simulink model "control_velocidades"  (Simulink 7.5)
settings: Solver=ode45  StartTime=0.0  StopTime=10.0  RelTol=1e-3
libraries: simulink x1
settings Model: Creator=ARTURO  LastModifiedBy=ARTURO

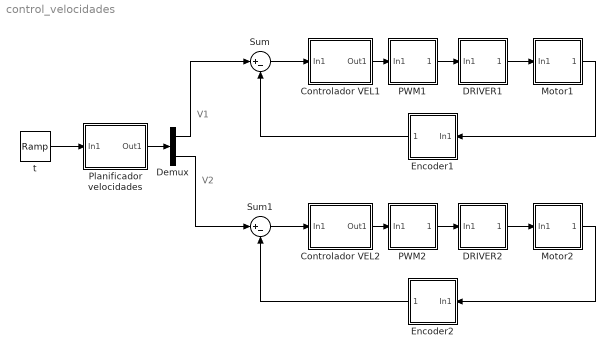
== system control_velocidades ==
  note: V1
  note: V2
  Controlador VEL1 : Subsystem
  Controlador VEL2 : Subsystem
  DRIVER1 : Subsystem
  DRIVER2 : Subsystem
  Demux : Demux  Outputs=2
  Encoder1 : Subsystem
  Encoder2 : Subsystem
  Motor1 : Subsystem
  Motor2 : Subsystem
  PWM1 : Subsystem
  PWM2 : Subsystem
  Planificador velocidades : Subsystem
  Sum : Sum  Inputs=|+-  OutDataType=fixdt(1, 16)  OutScaling=2^0
  Sum1 : Sum  Inputs=|+-  OutDataType=fixdt(1, 16)  OutScaling=2^0
  t : simulink/Sources/Ramp  SystemSampleTime=-1  slope=1  start=0  X0=0
  wires:
  Sum/1 -> Controlador VEL1/1(In1)
  Controlador VEL1/1(Out1) -> PWM1/1(In1)
  PWM1/1(Out1) -> DRIVER1/1(In1)
  DRIVER1/1(Out1) -> Motor1/1(In1)
  Motor1/1(Out1) -> Encoder1/1(In1)
  Encoder1/1(Out1) -> Sum/2
  Demux/1 -> Sum/1
  Sum1/1 -> Controlador VEL2/1(In1)
  Controlador VEL2/1(Out1) -> PWM2/1(In1)
  PWM2/1(Out1) -> DRIVER2/1(In1)
  DRIVER2/1(Out1) -> Motor2/1(In1)
  Motor2/1(Out1) -> Encoder2/1(In1)
  Encoder2/1(Out1) -> Sum1/2
  Demux/2 -> Sum1/1
  Planificador velocidades/1(Out1) -> Demux/1
  t/1 -> Planificador velocidades/1(In1)

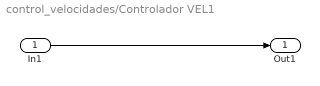
== system control_velocidades/Controlador VEL1 ==
  In1 : Inport  OutDataType=fixdt(1, 16)  OutScaling=2^0
  Out1 : Outport  OutDataType=fixdt(1, 16)  OutScaling=2^0
  wires:
  In1/1 -> Out1/1

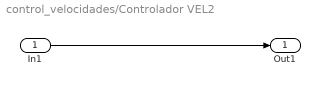
== system control_velocidades/Controlador VEL2 ==
  In1 : Inport  OutDataType=fixdt(1, 16)  OutScaling=2^0
  Out1 : Outport  OutDataType=fixdt(1, 16)  OutScaling=2^0
  wires:
  In1/1 -> Out1/1

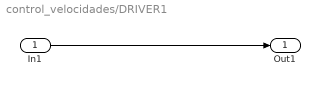
== system control_velocidades/DRIVER1 ==
  In1 : Inport  OutDataType=fixdt(1, 16)  OutScaling=2^0
  Out1 : Outport  OutDataType=fixdt(1, 16)  OutScaling=2^0
  wires:
  In1/1 -> Out1/1

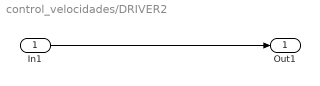
== system control_velocidades/DRIVER2 ==
  In1 : Inport  OutDataType=fixdt(1, 16)  OutScaling=2^0
  Out1 : Outport  OutDataType=fixdt(1, 16)  OutScaling=2^0
  wires:
  In1/1 -> Out1/1

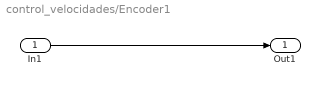
== system control_velocidades/Encoder1 ==
  In1 : Inport  OutDataType=fixdt(1, 16)  OutScaling=2^0
  Out1 : Outport  OutDataType=fixdt(1, 16)  OutScaling=2^0
  wires:
  In1/1 -> Out1/1

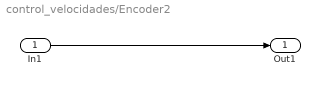
== system control_velocidades/Encoder2 ==
  In1 : Inport  OutDataType=fixdt(1, 16)  OutScaling=2^0
  Out1 : Outport  OutDataType=fixdt(1, 16)  OutScaling=2^0
  wires:
  In1/1 -> Out1/1

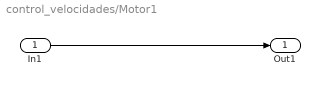
== system control_velocidades/Motor1 ==
  In1 : Inport  OutDataType=fixdt(1, 16)  OutScaling=2^0
  Out1 : Outport  OutDataType=fixdt(1, 16)  OutScaling=2^0
  wires:
  In1/1 -> Out1/1

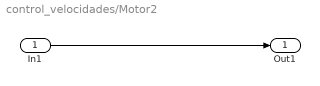
== system control_velocidades/Motor2 ==
  In1 : Inport  OutDataType=fixdt(1, 16)  OutScaling=2^0
  Out1 : Outport  OutDataType=fixdt(1, 16)  OutScaling=2^0
  wires:
  In1/1 -> Out1/1

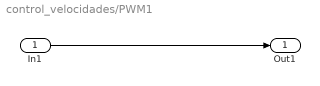
== system control_velocidades/PWM1 ==
  In1 : Inport  OutDataType=fixdt(1, 16)  OutScaling=2^0
  Out1 : Outport  OutDataType=fixdt(1, 16)  OutScaling=2^0
  wires:
  In1/1 -> Out1/1

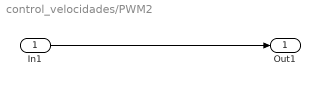
== system control_velocidades/PWM2 ==
  In1 : Inport  OutDataType=fixdt(1, 16)  OutScaling=2^0
  Out1 : Outport  OutDataType=fixdt(1, 16)  OutScaling=2^0
  wires:
  In1/1 -> Out1/1

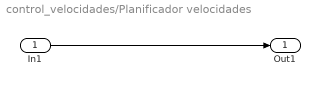
== system control_velocidades/Planificador velocidades ==
  In1 : Inport  OutDataType=fixdt(1, 16)  OutScaling=2^0
  Out1 : Outport  OutDataType=fixdt(1, 16)  OutScaling=2^0
  wires:
  In1/1 -> Out1/1
